simulink library "tetherM_cl"  (R2022a)
settings: Solver=VariableStepAuto  StartTime=0.0  StopTime=10.0  RelTol=1e-3
undefined symbols (not defined in the file): env, initNodePos, nodePosToLinkPos, nodePosToLinkPos_ul, numNodes, tetherReelSpeed, thr, vhcl
libraries: matrix_library x2, firstOrderFilter_ul x1
settings Model: Creator=mr-jo  LastModifiedBy=jbfine
settings SolverCC: AlgebraicLoopSolver=TrustRegion
settings DebuggingCC: UnconnectedInputMsg=warning  UnconnectedOutputMsg=warning  UnconnectedLineMsg=warning  SFMachineParentedDataDiag=warning

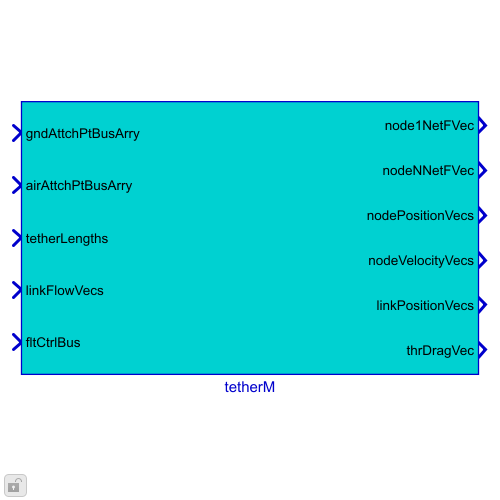
[thumbnail: Simulink's stored preview of the top-level diagram]
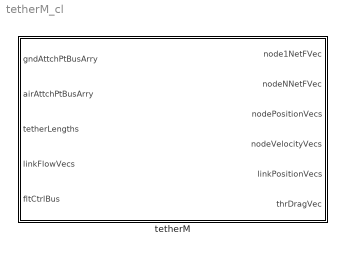
== system tetherM_cl ==
  tetherM : Subsystem  VariantControl=VSS_tethers_tetherM  mask{thr=thr, fluidDensity=env.water.density.Value, gravity=env.gravAccel.Value}
      mask prompts: thr "Tether001 Object"; fluidDensity "Fluid Density"; gravity "Gravitational Aceleration"

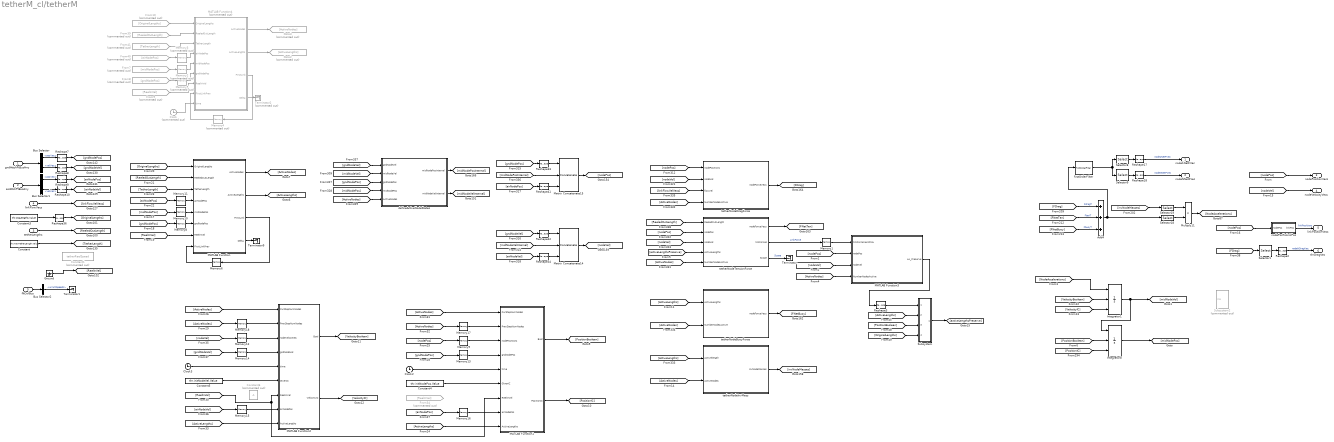
== system tetherM_cl/tetherM ==
  gndAttchPtBusArry : Inport  OutDataTypeStr=Bus: thrAttachPtKinematicsBus
  airAttchPtBusArry : Inport  Port=2  OutDataTypeStr=Bus: thrAttachPtKinematicsBus
  tetherLengths : Inport  Port=3
  linkFlowVecs : Inport  Port=4
  fltCtrlBus : Inport  Port=5
  Add4 : Sum  Inputs=3
  Bus Selector : BusSelector  OutputSignals=posVec,velVec
  Bus Selector1 : BusSelector  OutputSignals=posVec,velVec
  Bus Selector2 : BusSelector  OutputSignals=winchSpeeds
  Clock : Clock  Commented=on
  Clock2 : Clock
  Clock3 : Clock
  Constant : Constant  Value=thr.maxTetherLength.Value
  Constant1 : Constant  Commented=on  Value=tetherReelSpeed
  Constant3 : Constant  Value=thr.orgLengths.Value
  Constant4 : Constant  Value=thr.initNodePos.Value
  Constant5 : Constant  Value=thr.initNodeVel.Value
  Constant6 : Constant  Commented=on  Value=-1
  From10 : From  Commented=on  GotoTag=OriginalLengths
  From34 : From  Commented=on  GotoTag=ReelInVel
  From39 : From  Commented=on  GotoTag=ReeledOutLength
  From40 : From  Commented=on  GotoTag=airNodePos
  From41 : From  Commented=on  GotoTag=TetherLength
  From7 : From  Commented=on  GotoTag=midNodePos
  From8 : From  Commented=on  GotoTag=gndNodePos
  From9 : From  Commented=on  GotoTag=ReelInVel
  Goto2 : Goto  Commented=on  GotoTag=ActiveLengths
  Goto3 : Goto  Commented=on  GotoTag=ActiveNodes
  Ground : Ground
  Integrator1 : Integrator  ExternalReset=rising  InitialConditionSource=external
  Integrator8 : Integrator  ExternalReset=rising  InitialConditionSource=external
  MATLAB Function : MATLAB Function  TreatAsAtomicUnit=on  mask{minLinkLength=thr.minLinkLength.Value, minLinkDeviation=thr.minLinkDeviation.Value}
      mask prompts: minLinkLength "Minimum Link Length"; minLinkDeviation "Minimum Devation to Remove Node"
  MATLAB Function1 : MATLAB Function  TreatAsAtomicUnit=on
  MATLAB Function2 : MATLAB Function  TreatAsAtomicUnit=on
  MATLAB Function3 : MATLAB Function  TreatAsAtomicUnit=on  mask{numNodes=thr.numNodes.Value, thrDiam=thr.diameter.Value, youngsMod=thr.youngsMod.Value, dampingRatio=thr.dampingRatio.Value, mass=vhcl.mass.Value}
      mask prompts: numNodes "Number of Nodes"; thrDiam "Tether Diameter"; youngsMod "Youngs Mod of Tether"; dampingRatio "Total Tether Damping Ratio"; mass "Vehicle Mass for Damping"
  MATLAB Function4 : MATLAB Function  Commented=on  TreatAsAtomicUnit=on  mask{minLinkLength=thr.minLinkLength.Value, minLinkDeviation=thr.minLinkDeviation.Value}
      mask prompts: minLinkLength "Minimum Link Length"; minLinkDeviation "Minimum Devation to Remove Node"
  Matrix Concatenate14 : Concatenate  NumInputs=3  Mode=Multidimensional array  ConcatenateDimension=2
  Matrix Concatenate15 : Concatenate  NumInputs=3  Mode=Multidimensional array  ConcatenateDimension=2
  Memory{1,6,8..18} (13 alike) : Memory
  Memory{2..5} (4 alike) : Memory  Commented=on
  Multiply11 : Product
  Reshape{2,7..10,17..18,33..34,41..42} (11 alike) : Reshape  OutputDimensionality=Column vector (2-D)
  Reshape3 : Reshape  OutputDimensionality=Row vector (2-D)
  Reshape36 : Reshape  OutputDimensionality=Row vector (2-D)
  Selector1 : Selector  NumberOfDimensions=2  InputPortWidth=3  IndexOptions=Select all,Starting index (dialog)  Indices=[1 3],thr.numNodes.Value  OutputSizes=1,1
  Selector18 : Selector  NumberOfDimensions=2  InputPortWidth=3  IndexOptions=Select all,Index vector (dialog)  Indices=[1 3],2:thr.numNodes.Value-1  OutputSizes=1,1
  Selector19 : Selector  NumberOfDimensions=2  InputPortWidth=3  IndexOptions=Select all,Index vector (dialog)  Indices=[1 3],2:thr.numNodes.Value-1  OutputSizes=1,1
  Selector8 : Selector  NumberOfDimensions=2  InputPortWidth=3  IndexOptions=Select all,Index vector (dialog)  Indices=[1 3],1  OutputSizes=1,1
  Selector9 : Selector  NumberOfDimensions=2  InputPortWidth=3  IndexOptions=Select all,Starting index (dialog)  Indices=[1 3],thr.numNodes.Value  OutputSizes=1,1
  Subsystem : Subsystem
  Subsystem2 : Subsystem  Commented=on
  Terminator : Terminator
  Terminator1 : Terminator
  Terminator2 : Terminator  Commented=on
  Terminator9 : Terminator
  defineActiveNodeStates : MATLAB Function  TreatAsAtomicUnit=on
  firstOrderFilter : firstOrderFilter_ul/firstOrderFilter  tau=0.1  ic=0
  nodePosToLinkPos : Subsystem  AncestorBlock=nodePosToLinkPos_ul/nodePosToLinkPos
  tetherNodeBuoyForce : MATLAB Function  TreatAsAtomicUnit=on  mask{fluidDensity=fluidDensity, numNodes=thr.numNodes.Value, thrDiam=thr.diameter.Value, tetherDensity=thr.density.Value, gravity=gravity}
      mask prompts: fluidDensity "Fluid Density"; numNodes "Number of Nodes"; thrDiam "Tether Diameter"; tetherDensity "Tether Density"; gravity "Gravitational Acceleration"
  tetherNodeDragForce : MATLAB Function  TreatAsAtomicUnit=on  mask{flowDensity=fluidDensity, numNodes=thr.numNodes.Value, dragCoeff=thr.dragCoeff.Value, thrDiam=thr.diameter.Value}
      mask prompts: flowDensity "Fluid Density"; numNodes "Number of nodes"; dragCoeff "Drag Coefficient of Tether"; thrDiam "Tether Diameter"
  tetherNodeInvMass : MATLAB Function  TreatAsAtomicUnit=on  mask{numNodes=thr.numNodes.Value, thrDiam=thr.diameter.Value, tetherDensity=thr.density.Value}
      mask prompts: numNodes "Number of nodes"; thrDiam "Tether Diameter"; tetherDensity "Tether Density"
  tetherNodeTensionForce : MATLAB Function  TreatAsAtomicUnit=on  mask{numNodes=thr.numNodes.Value, thrDiam=thr.diameter.Value, youngsMod=thr.youngsMod.Value, dampingRatio=thr.dampingRatio.Value, mass=vhcl.mass.Value, minSoftLength=thr.minSoftLength.Value}
      mask prompts: numNodes "Number of Nodes"; thrDiam "Tether Diameter"; youngsMod "Youngs Modulus of Tether"; dampingRatio "Total Tether Damping Ratio"; mass "Vehicle Mass for Damping"; minSoftLength "Min Link Length for Spring Softening"
  node1NetFVec : Outport  VectorParamsAs1DForOutWhenUnconnected=off
  nodeNNetFVec : Outport  Port=2  VectorParamsAs1DForOutWhenUnconnected=off
  nodePositionVecs : Outport  Port=3  VectorParamsAs1DForOutWhenUnconnected=off
  nodeVelocityVecs : Outport  Port=4  VectorParamsAs1DForOutWhenUnconnected=off
  linkPositionVecs : Outport  Port=5  VectorParamsAs1DForOutWhenUnconnected=off
  thrDragVec : Outport  Port=6  VectorParamsAs1DForOutWhenUnconnected=off
  wires:
  Ground/1 -> [ReelInVel]
  [activeLengthsPreserve] -> tetherNodeTensionForce/4(ActiveLengths)
  Integrator1/1 -> Integrator8/1, [midNodeVel]
  [NodeAccelerations] -> Integrator1/1
  Integrator8/1 -> [midNodePos]
  Clock/1 -> MATLAB Function4/9(time)
  From39/1 -> MATLAB Function4/2(ReeledOutLength)
  MATLAB Function4/1(ActiveNodes) -> Goto3/1
  Memory3/1 -> MATLAB Function4/4(airNodePos)
  From40/1 -> Memory3/1
  MATLAB Function4/3(FirstLink) -> Memory4/1
  Memory2/1 -> MATLAB Function4/5(midNodePos)
  From7/1 -> Memory2/1
  MATLAB Function4/4(Delta) -> Terminator2/1
  From8/1 -> Memory5/1
  Memory5/1 -> MATLAB Function4/6(gndNodePos)
  MATLAB Function4/2(ActiveLengths) -> Goto2/1
  From9/1 -> MATLAB Function4/7(ReelInVel)
  From41/1 -> MATLAB Function4/3(TetherLength)
  From10/1 -> MATLAB Function4/1(OriginalLengths)
  Memory4/1 -> MATLAB Function4/8(FirstLinkPrev)
  MATLAB Function3/1(LA_Preserve) -> Reshape3/1
  tetherNodeTensionForce/2(linkForces) -> Memory1/1  "LinkForce"
  Memory1/1 -> MATLAB Function3/1(linkForceVecsPrev)
  [ActiveNodes] -> MATLAB Function3/4(NumberNodesActive)
  [nodeVel] -> MATLAB Function3/3(nodeVel)
  [nodePos] -> MATLAB Function3/2(nodePos)
  Reshape3/1 -> Subsystem/1(In1)
  [OriginalLengths] -> Subsystem/4(In4)
  [PositionBoolean] -> Subsystem/3(In3)
  [ActiveLengths] -> Subsystem/2(In2)
  Subsystem/1(Out1) -> [activeLengthsPreserve]
  MATLAB Function/4(Delta) -> Terminator9/1
  tetherNodeTensionForce/3(Scope) -> Terminator/1  "Scope"
  [nodeVel] -> tetherNodeTensionForce/3(nodeVel)
  [nodeVel] -> tetherNodeDragForce/2(nodeVel)
  [ReelInVel] -> MATLAB Function1/7(ReelInVel), MATLAB Function2/7(ReelInVel)
  Reshape2/1 -> thrDragVec/1  "nodeNDragVec"
  [FDrag] -> Selector1/1
  Selector1/1 -> Reshape2/1
  Selector18/1 -> Multiply11/2
  Add4/1 -> firstOrderFilter/1, Selector18/1
  firstOrderFilter/1 -> Selector8/1, Selector9/1
  [FNetTen] -> Add4/2  "FtenT"
  Reshape18/1 -> nodeNNetFVec/1  "nodeNNetFVec"
  Reshape17/1 -> node1NetFVec/1  "node1NetFVec"
  [ActiveNodes] -> Memory18/1
  [ActiveNodes] -> Memory17/1
  Constant4/1 -> MATLAB Function1/6(GivenIC)
  MATLAB Function1/1(Bool) -> [PositionBoolean]
  [ActiveNodes] -> MATLAB Function2/1(CurStepNumNodes)
  Memory16/1 -> MATLAB Function1/8(airNodePos)
  Clock2/1 -> MATLAB Function1/5(time)
  MATLAB Function2/2(VelocityIC) -> [VelocityIC]
  Memory13/1 -> MATLAB Function1/4(gndNodePos)
  [airNodeVel] -> Memory15/1
  MATLAB Function1/2(PositionIC) -> [PositionIC]
  Clock3/1 -> MATLAB Function2/5(time)
  [gndNodePos] -> Memory13/1
  Memory17/1 -> MATLAB Function1/2(PrevStepNumNodes)
  [nodeVel] -> Memory12/1
  [gndNodeVel] -> Memory14/1
  Memory18/1 -> MATLAB Function2/2(PrevStepNumNodes)
  Constant5/1 -> MATLAB Function2/6(GivenIC)
  Memory14/1 -> MATLAB Function2/4(gndNodeVel)
  [nodePos] -> Memory9/1
  [ActiveLengths] -> MATLAB Function1/9(ActiveLengths)
  [ActiveNodes] -> MATLAB Function1/1(CurStepNumNodes)
  Memory15/1 -> MATLAB Function2/8(airNodePos)
  [airNodePos] -> Memory16/1
  Memory9/1 -> MATLAB Function1/3(nodePositions)
  MATLAB Function2/1(Bool) -> [VelocityBoolean]
  Memory12/1 -> MATLAB Function2/3(nodeVelocities)
  [ActiveLengths] -> MATLAB Function2/9(ActiveLengths)
  MATLAB Function/2(ActiveLengths) -> [ActiveLengths]
  [midNodePos] -> Memory10/1
  MATLAB Function/1(ActiveNodes) -> [ActiveNodes]
  [ReeledOutLength] -> MATLAB Function/2(ReeledOutLength)
  [ReelInVel] -> MATLAB Function/7(ReelInVel)
  [OriginalLengths] -> MATLAB Function/1(OriginalLengths)
  [airNodePos] -> Memory11/1
  [TetherLength] -> MATLAB Function/3(TetherLength)
  MATLAB Function/3(FirstLink) -> Memory6/1
  Memory8/1 -> MATLAB Function/6(gndNodePos)
  Memory10/1 -> MATLAB Function/5(midNodePos)
  Memory11/1 -> MATLAB Function/4(airNodePos)
  Memory6/1 -> MATLAB Function/8(FirstLinkPrev)
  [gndNodePos] -> Memory8/1
  tetherNodeDragForce/1(nodeForceVecs) -> [FDrag]
  [gndNodeVel] -> Reshape42/1
  [ActiveNodes] -> tetherNodeTensionForce/5(NumberNodesActive)
  tetherNodeInvMass/1(invNodeMasses) -> [invNodeMasses]
  [gndNodePos] -> Reshape33/1
  [airNodePos] -> Reshape41/1
  [midNodePosInternal] -> Matrix Concatenate15/2
  [nodePos] -> tetherNodeDragForce/1(nodePositions)
  [ActiveLengths] -> tetherNodeInvMass/1(Activelength)
  tetherNodeBuoyForce/1(nodeForceVecs) -> [FNetBuoy]
  Reshape42/1 -> Matrix Concatenate14/1
  [ActiveNodes] -> tetherNodeBuoyForce/2(NumberNodesActive)
  Reshape41/1 -> Matrix Concatenate15/3
  Reshape33/1 -> Matrix Concatenate15/1
  [airNodeVel] -> Reshape34/1
  Matrix Concatenate14/1 -> [nodeVel]
  tetherNodeTensionForce/1(nodeForceVecs) -> [FNetTen]
  Matrix Concatenate15/1 -> [nodePos]
  [gndNodeVel] -> defineActiveNodeStates/1(gndNodeVel)
  [midNodePos] -> defineActiveNodeStates/4(midNodePos)
  [ActiveNodes] -> defineActiveNodeStates/5(ActiveNodes)
  [midNodeVelInternal] -> Matrix Concatenate14/2
  [gndNodePos] -> defineActiveNodeStates/3(gndNodePos)
  Reshape34/1 -> Matrix Concatenate14/3
  [ActiveNodes] -> tetherNodeDragForce/4(NumberNodesActive)
  [ReeledOutLength] -> tetherNodeTensionForce/1(ReeledOutLength)
  defineActiveNodeStates/2(midNodeVelInternal) -> [midNodeVelInternal]
  [nodePos] -> tetherNodeTensionForce/2(nodePos)
  [midNodeVel] -> defineActiveNodeStates/2(midNodeVel)
  [linkFlowVelVecs] -> tetherNodeDragForce/3(flowVel)
  tetherLengths/1 -> [ReeledOutLength]
  Reshape36/1 -> [OriginalLengths]
  linkFlowVecs/1 -> [linkFlowVelVecs]
  Constant/1 -> [TetherLength]
  defineActiveNodeStates/1(midNodePosInternal) -> [midNodePosInternal]
  [invNodeMasses] -> Selector19/1
  Selector19/1 -> Multiply11/1
  [FDrag] -> Add4/1  "FdragT"
  Multiply11/1 -> [NodeAccelerations]
  [FNetBuoy] -> Add4/3  "FbuoyT"
  [PositionIC] -> Integrator8/3
  Selector8/1 -> Reshape17/1
  Selector9/1 -> Reshape18/1
  [PositionBoolean] -> Integrator8/2
  [VelocityIC] -> Integrator1/3
  [VelocityBoolean] -> Integrator1/2
  [ActiveLengths] -> tetherNodeBuoyForce/1(ActiveLengths)
  [ActiveNodes] -> tetherNodeInvMass/2(ActiveNodes)
  Bus Selector1/2 -> Reshape10/1  "<velVec>"
  gndAttchPtBusArry/1 -> Bus Selector/1
  Reshape7/1 -> [gndNodePos]
  Reshape10/1 -> [airNodeVel]
  Reshape9/1 -> [airNodePos]
  airAttchPtBusArry/1 -> Bus Selector1/1
  Bus Selector/2 -> Reshape8/1  "<velVec>"
  Bus Selector1/1 -> Reshape9/1  "<posVec>"
  Reshape8/1 -> [gndNodeVel]
  Bus Selector/1 -> Reshape7/1  "<posVec>"
  Constant3/1 -> Reshape36/1
  [nodePos] -> nodePositionVecs/1
  [nodeVel] -> nodeVelocityVecs/1
  nodePosToLinkPos/1("linkPos ") -> linkPositionVecs/1  "linkPositions"
  [nodePos] -> nodePosToLinkPos/1("nodePos ")
  fltCtrlBus/1 -> Bus Selector2/1
  Bus Selector2/1 -> Terminator1/1  "<winchSpeeds>"

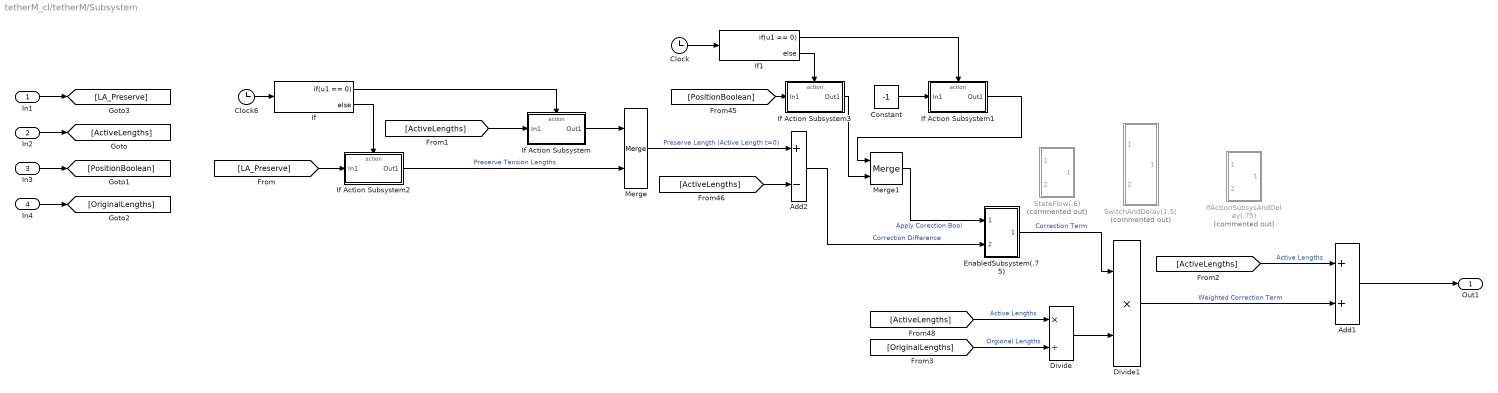
== system tetherM_cl/tetherM/Subsystem ==
  In1 : Inport
  In2 : Inport  Port=2
  In3 : Inport  Port=3
  In4 : Inport  Port=4
  Add1 : Sum
  Add2 : Sum  Inputs=+-
  Clock : Clock
  Clock6 : Clock
  Constant : Constant  Value=-1
  Divide : Product  Inputs=*/
  Divide1 : Product  Inputs=**
  EnabledSubsystem(.75) : Subsystem
  If : If  IfExpression=u1 == 0
  If Action Subsystem : Subsystem  TreatAsAtomicUnit=on
  If Action Subsystem1 : Subsystem  TreatAsAtomicUnit=on
  If Action Subsystem2 : Subsystem  TreatAsAtomicUnit=on
  If Action Subsystem3 : Subsystem  TreatAsAtomicUnit=on
  If1 : If  IfExpression=u1 == 0
  IfActionSubsysAndDelay(.75) : Subsystem  Commented=on
  Merge : Merge  InitialOutput=thr.orgLengths.Value
  Merge1 : Merge  InitialOutput=[-1]
  StateFlow(.6) : Subsystem  Commented=on
  SwitchAndDelay(1.5) : Subsystem  Commented=on
  Out1 : Outport
  wires:
  Add1/1 -> Out1/1
  [ActiveLengths] -> Add1/1  "Active Lengths"
  [ActiveLengths] -> Divide/1  "Active Lengths"
  [ActiveLengths] -> Add2/2
  [ActiveLengths] -> If Action Subsystem/1(In1)
  If Action Subsystem1/1(Out1) -> Merge1/1
  Constant/1 -> If Action Subsystem1/1(In1)
  If Action Subsystem3/1(Out1) -> Merge1/2
  Merge1/1 -> EnabledSubsystem(.75)/1(Enable)  "Apply Corection Bool"
  If1/2 -> If Action Subsystem3/Action
  If1/1 -> If Action Subsystem1/Action
  Clock/1 -> If1/1
  EnabledSubsystem(.75)/1(Out1) -> Divide1/1  "Correction Term"
  Add2/1 -> EnabledSubsystem(.75)/2(In2)  "Correction Difference"
  [PositionBoolean] -> If Action Subsystem3/1(In1)
  Merge/1 -> Add2/1  "Preserve Length (Active Length t=0)"
  [LA_Preserve] -> If Action Subsystem2/1(In1)
  In4/1 -> [OriginalLengths]
  In3/1 -> [PositionBoolean]
  In2/1 -> [ActiveLengths]
  In1/1 -> [LA_Preserve]
  If/1 -> If Action Subsystem/Action
  Divide/1 -> Divide1/2
  If/2 -> If Action Subsystem2/Action
  If Action Subsystem/1(Out1) -> Merge/1
  [OriginalLengths] -> Divide/2  "Orgional Lengths"
  If Action Subsystem2/1(Out1) -> Merge/2  "Preserve Tension Lengths"
  Clock6/1 -> If/1
  Divide1/1 -> Add1/2  "Weighted Correction Term"

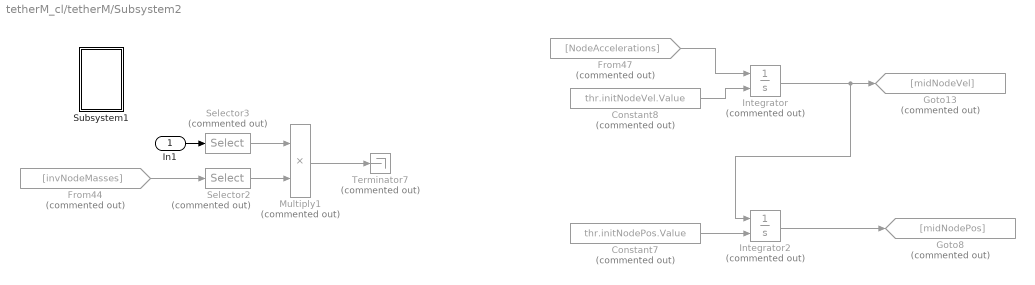
== system tetherM_cl/tetherM/Subsystem2 ==
  In1 : Inport
  Constant7 : Constant  Commented=on  Value=thr.initNodePos.Value
  Constant8 : Constant  Commented=on  Value=thr.initNodeVel.Value
  From44 : From  Commented=on  GotoTag=invNodeMasses
  From47 : From  Commented=on  GotoTag=NodeAccelerations
  Goto13 : Goto  Commented=on  GotoTag=midNodeVel
  Goto8 : Goto  Commented=on  GotoTag=midNodePos
  Integrator : Integrator  Commented=on  InitialConditionSource=external
  Integrator2 : Integrator  Commented=on  InitialConditionSource=external
  Multiply1 : Product  Commented=on
  Selector2 : Selector  Commented=on  NumberOfDimensions=2  InputPortWidth=3  IndexOptions=Select all,Index vector (dialog)  Indices=[1 3],2:thr.numNodes.Value-1  OutputSizes=1,1
  Selector3 : Selector  Commented=on  NumberOfDimensions=2  InputPortWidth=3  IndexOptions=Select all,Index vector (dialog)  Indices=[1 3],2:thr.numNodes.Value-1  OutputSizes=1,1
  Subsystem1 : Subsystem
  Terminator7 : Terminator  Commented=on
  wires:
  In1/1 -> Selector3/1
  Selector2/1 -> Multiply1/2
  From44/1 -> Selector2/1
  Integrator2/1 -> Goto8/1
  Constant8/1 -> Integrator/2
  Multiply1/1 -> Terminator7/1
  From47/1 -> Integrator/1
  Constant7/1 -> Integrator2/2
  Integrator/1 -> Goto13/1, Integrator2/1
  Selector3/1 -> Multiply1/1

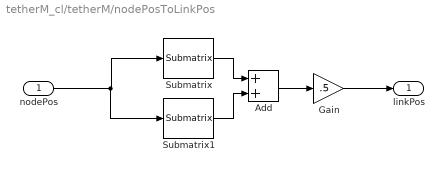
== system tetherM_cl/tetherM/nodePosToLinkPos ==
  "nodePos " : Inport
  Add : Sum
  Gain : Gain  Gain=.5
  Submatrix : matrix_library/Submatrix  RowSpan=All rows  RowStartMode=First  RowStartIndex=1  RowEndMode=Last  RowEndIndex=1  ColSpan=Range of columns  ColStartMode=First  ColStartIndex=1  ColEndMode=Offset from last  ColEndIndex=1
      settings: SourceProductBaseCode=SL
  Submatrix1 : matrix_library/Submatrix  RowSpan=All rows  RowStartMode=First  RowStartIndex=1  RowEndMode=Last  RowEndIndex=1  ColSpan=Range of columns  ColStartMode=Index  ColStartIndex=2  ColEndMode=Last  ColEndIndex=1
      settings: SourceProductBaseCode=SL
  "linkPos " : Outport  VectorParamsAs1DForOutWhenUnconnected=off
  wires:
  "nodePos "/1 -> Submatrix1/1, Submatrix/1
  Gain/1 -> "linkPos "/1
  Add/1 -> Gain/1
  Submatrix/1 -> Add/1
  Submatrix1/1 -> Add/2

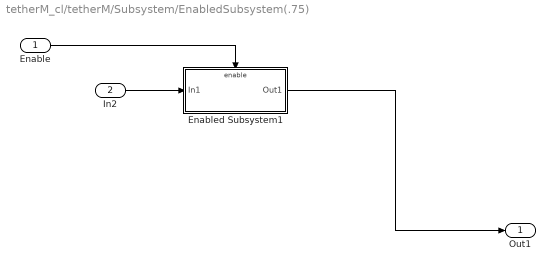
== system tetherM_cl/tetherM/Subsystem/EnabledSubsystem(.75) ==
  Enable : Inport
  In2 : Inport  Port=2
  Enabled Subsystem1 : Subsystem  TreatAsAtomicUnit=on
  Out1 : Outport
  wires:
  In2/1 -> Enabled Subsystem1/1(In1)
  Enabled Subsystem1/1(Out1) -> Out1/1
  Enable/1 -> Enabled Subsystem1/Enable

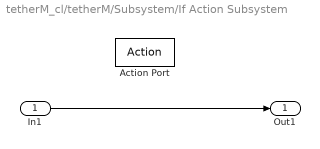
== system tetherM_cl/tetherM/Subsystem/If Action Subsystem ==
  In1 : Inport
  Action Port : ActionPort
  Out1 : Outport
  wires:
  In1/1 -> Out1/1

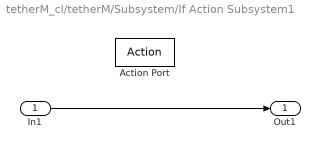
== system tetherM_cl/tetherM/Subsystem/If Action Subsystem1 ==
  In1 : Inport
  Action Port : ActionPort
  Out1 : Outport
  wires:
  In1/1 -> Out1/1

== system tetherM_cl/tetherM/Subsystem/If Action Subsystem2 ==
  In1 : Inport
  Action Port : ActionPort
  Out1 : Outport
  wires:
  In1/1 -> Out1/1

== system tetherM_cl/tetherM/Subsystem/If Action Subsystem3 ==
  In1 : Inport
  Action Port : ActionPort
  Out1 : Outport
  wires:
  In1/1 -> Out1/1

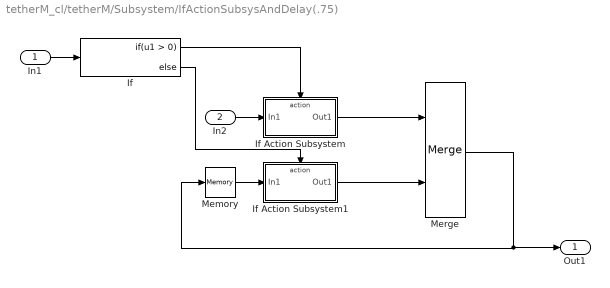
== system tetherM_cl/tetherM/Subsystem/IfActionSubsysAndDelay(.75) ==
  In1 : Inport
  In2 : Inport  Port=2
  If : If
  If Action Subsystem : Subsystem  TreatAsAtomicUnit=on
  If Action Subsystem1 : Subsystem  TreatAsAtomicUnit=on
  Memory : Memory
  Merge : Merge  InitialOutput=thr.orgLengths.Value
  Out1 : Outport
  wires:
  In2/1 -> If Action Subsystem/1(In1)
  In1/1 -> If/1
  Merge/1 -> Memory/1, Out1/1
  Memory/1 -> If Action Subsystem1/1(In1)
  If Action Subsystem1/1(Out1) -> Merge/2
  If Action Subsystem/1(Out1) -> Merge/1
  If/1 -> If Action Subsystem/Action
  If/2 -> If Action Subsystem1/Action

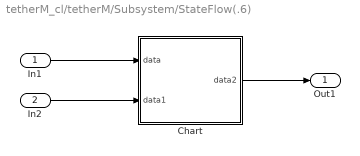
== system tetherM_cl/tetherM/Subsystem/StateFlow(.6) ==
  In1 : Inport
  In2 : Inport  Port=2
  Chart : Stateflow chart  TreatAsAtomicUnit=on
  Out1 : Outport
  wires:
  Chart/1(data2) -> Out1/1
  In2/1 -> Chart/2(data1)
  In1/1 -> Chart/1(data)

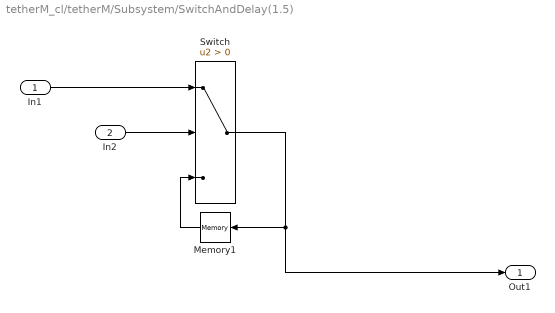
== system tetherM_cl/tetherM/Subsystem/SwitchAndDelay(1.5) ==
  In1 : Inport
  In2 : Inport  Port=2
  Memory1 : Memory  InitialCondition=zeros(size(thr.orgLengths.Value))
  Switch : Switch  Criteria=u2 > Threshold  SaturateOnIntegerOverflow=off  InputSameDT=off
  Out1 : Outport
  wires:
  In1/1 -> Switch/1
  In2/1 -> Switch/2
  Memory1/1 -> Switch/3
  Switch/1 -> Memory1/1, Out1/1

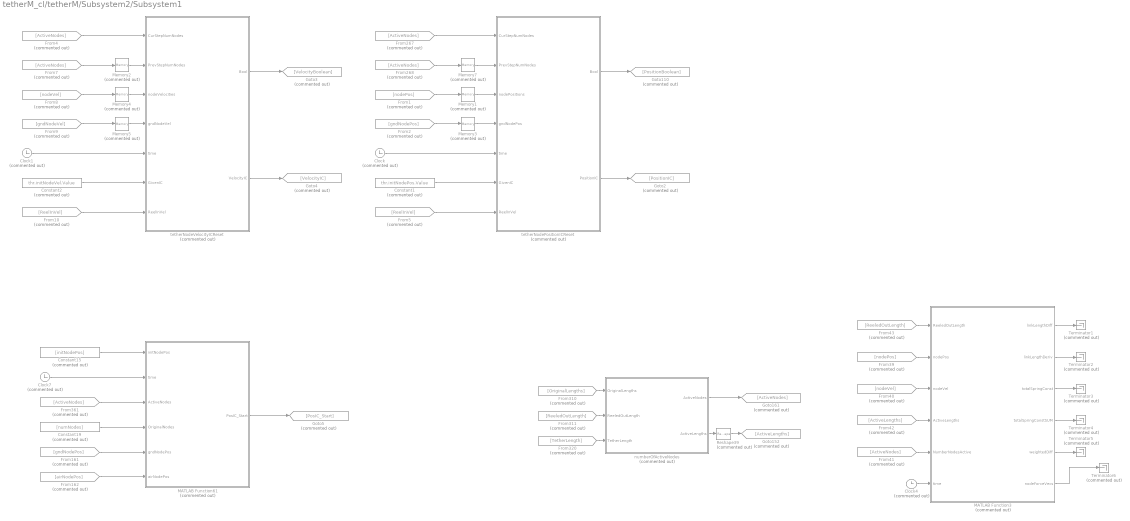
== system tetherM_cl/tetherM/Subsystem2/Subsystem1 ==
  Clock{,1,4,7} (4 alike) : Clock  Commented=on
  Constant1 : Constant  Commented=on  Value=thr.initNodePos.Value
  Constant15 : Constant  Commented=on  Value=[initNodePos]
  Constant19 : Constant  Commented=on  Value=[numNodes]
  Constant2 : Constant  Commented=on  Value=thr.initNodeVel.Value
  From1 : From  Commented=on  GotoTag=nodePos
  From10 : From  Commented=on  GotoTag=ReelInVel
  From161 : From  Commented=on  GotoTag=gndNodePos
  From162 : From  Commented=on  GotoTag=airNodePos
  From2 : From  Commented=on  GotoTag=gndNodePos
  From{4,7,41,267..268,361} (6 alike) : From  Commented=on  GotoTag=ActiveNodes
  From310 : From  Commented=on  GotoTag=OriginalLengths
  From311 : From  Commented=on  GotoTag=ReeledOutLength
  From320 : From  Commented=on  GotoTag=TetherLength
  From39 : From  Commented=on  GotoTag=nodePos
  From40 : From  Commented=on  GotoTag=nodeVel
  From42 : From  Commented=on  GotoTag=ActiveLengths
  From43 : From  Commented=on  GotoTag=ReeledOutLength
  From5 : From  Commented=on  GotoTag=ReelInVel
  From8 : From  Commented=on  GotoTag=nodeVel
  From9 : From  Commented=on  GotoTag=gndNodeVel
  Goto110 : Goto  Commented=on  GotoTag=PositionBoolean
  Goto152 : Goto  Commented=on  GotoTag=ActiveLengths
  Goto161 : Goto  Commented=on  GotoTag=ActiveNodes
  Goto2 : Goto  Commented=on  GotoTag=PositionIC
  Goto3 : Goto  Commented=on  GotoTag=VelocityBoolean
  Goto4 : Goto  Commented=on  GotoTag=VelocityIC
  Goto5 : Goto  Commented=on  GotoTag=PosIC_Start
  MATLAB Function3 : MATLAB Function  Commented=on  TreatAsAtomicUnit=on  mask{numNodes=thr.numNodes.Value, thrDiam=thr.diameter.Value, youngsMod=thr.youngsMod.Value, dampingRatio=thr.dampingRatio.Value, mass=thr.vehicleMass.Value}
      mask prompts: numNodes "Number of Nodes"; thrDiam "Tether Diameter"; youngsMod "Youngs Modulus of Tether"; dampingRatio "Total Tether Damping Ratio"; mass "Vehicle Mass for Damping"
  MATLAB Function61 : MATLAB Function  Commented=on  TreatAsAtomicUnit=on
  Memory{1..5,7} (6 alike) : Memory  Commented=on
  Reshape39 : Reshape  Commented=on  OutputDimensionality=Row vector (2-D)
  Terminator{1..6} (6 alike) : Terminator  Commented=on
  numberOfActiveNodes : MATLAB Function  Commented=on  TreatAsAtomicUnit=on
  tetherNodePositionICReset : MATLAB Function  Commented=on  TreatAsAtomicUnit=on
  tetherNodeVelocityICReset : MATLAB Function  Commented=on  TreatAsAtomicUnit=on
  wires:
  numberOfActiveNodes/2(ActiveLengths) -> Reshape39/1
  MATLAB Function61/1(PosIC_Start) -> Goto5/1
  From311/1 -> numberOfActiveNodes/2(ReeledOutLength)
  From268/1 -> Memory7/1
  tetherNodePositionICReset/2(PositionIC) -> Goto2/1
  From310/1 -> numberOfActiveNodes/1(OriginalLengths)
  From2/1 -> Memory3/1
  From10/1 -> tetherNodeVelocityICReset/7(ReelInVel)
  From4/1 -> tetherNodeVelocityICReset/1(CurStepNumNodes)
  tetherNodeVelocityICReset/2(VelocityIC) -> Goto4/1
  From320/1 -> numberOfActiveNodes/3(TetherLength)
  From5/1 -> tetherNodePositionICReset/7(ReelInVel)
  Clock1/1 -> tetherNodeVelocityICReset/5(time)
  From8/1 -> Memory4/1
  Constant1/1 -> tetherNodePositionICReset/6(GivenIC)
  Clock7/1 -> MATLAB Function61/2(time)
  From162/1 -> MATLAB Function61/6(airNodePos)
  Memory3/1 -> tetherNodePositionICReset/4(gndNodePos)
  Constant19/1 -> MATLAB Function61/4(OriginalNodes)
  MATLAB Function3/1(linkLengthDiff) -> Terminator1/1
  From161/1 -> MATLAB Function61/5(gndNodePos)
  MATLAB Function3/5(weightedDiff) -> Terminator5/1
  Constant2/1 -> tetherNodeVelocityICReset/6(GivenIC)
  tetherNodePositionICReset/1(Bool) -> Goto110/1
  MATLAB Function3/6(nodeForceVecs) -> Terminator6/1
  From9/1 -> Memory5/1
  Memory5/1 -> tetherNodeVelocityICReset/4(gndNodeVel)
  Memory7/1 -> tetherNodePositionICReset/2(PrevStepNumNodes)
  From7/1 -> Memory2/1
  numberOfActiveNodes/1(ActiveNodes) -> Goto161/1
  Clock/1 -> tetherNodePositionICReset/5(time)
  Memory1/1 -> tetherNodePositionICReset/3(nodePositions)
  Clock4/1 -> MATLAB Function3/6(time)
  Reshape39/1 -> Goto152/1
  From43/1 -> MATLAB Function3/1(ReeledOutLength)
  MATLAB Function3/2(linkLengthDeriv) -> Terminator2/1
  From267/1 -> tetherNodePositionICReset/1(CurStepNumNodes)
  MATLAB Function3/4(totalSpringConstSUM) -> Terminator4/1
  Memory4/1 -> tetherNodeVelocityICReset/3(nodeVelocities)
  From41/1 -> MATLAB Function3/5(NumberNodesActive)
  From1/1 -> Memory1/1
  MATLAB Function3/3(totalSpringConst) -> Terminator3/1
  From42/1 -> MATLAB Function3/4(ActiveLengths)
  tetherNodeVelocityICReset/1(Bool) -> Goto3/1
  From361/1 -> MATLAB Function61/3(ActiveNodes)
  From39/1 -> MATLAB Function3/2(nodePos)
  Memory2/1 -> tetherNodeVelocityICReset/2(PrevStepNumNodes)
  From40/1 -> MATLAB Function3/3(nodeVel)
  Constant15/1 -> MATLAB Function61/1(initNodePos)

== system tetherM_cl/tetherM/Subsystem/EnabledSubsystem(.75)/Enabled Subsystem1 ==
  In1 : Inport
  Enable : EnablePort
  Out1 : Outport  InitialOutput=zeros(size(thr.orgLengths.Value))
  wires:
  In1/1 -> Out1/1

== system tetherM_cl/tetherM/Subsystem/IfActionSubsysAndDelay(.75)/If Action Subsystem ==
  In1 : Inport
  Action Port : ActionPort
  Out1 : Outport
  wires:
  In1/1 -> Out1/1

== system tetherM_cl/tetherM/Subsystem/IfActionSubsysAndDelay(.75)/If Action Subsystem1 ==
  In1 : Inport
  Action Port : ActionPort
  Out1 : Outport
  wires:
  In1/1 -> Out1/1

== stateflow chart tetherM_cl/tetherM/Subsystem/StateFlow(.6)/Chart ==
  (default) -> (junction 4) : [data>0]{data2=data1;}
  data: data input; data1 input; data2 output

== matlab function tetherM_cl/tetherM/Subsystem2/Subsystem1/MATLAB Function3 ==
  data: ReeledOutLength input; linkLengthDiff output; nodePos input; linkLengthDeriv output; totalSpringConst output; nodeVel input; ActiveLengths input; NumberNodesActive input; time input; numNodes parameter; totalSpringConstSUM output; thrDiam parameter; youngsMod parameter; dampingRatio parameter; mass parameter; weightedDiff output; nodeForceVecs output
function [linkLengthDiff,linkLengthDeriv,totalSpringConst,totalSpringConstSUM,weightedDiff,nodeForceVecs] = fcn(ReeledOutLength, nodePos,nodeVel,ActiveLengths,NumberNodesActive,time, numNodes, thrDiam, youngsMod, dampingRatio, mass)

No = numNodes;
Na = NumberNodesActive;

unstretchedLength = ReeledOutLength; %Total Reeled out length

%finds vectors between nodes
linkVecs  = diff(nodePos,1,2);
linkLength = sqrt(sum(linkVecs.^2));

%Finds unit vectors between nodes
linkUnitVecs = zeros(3,numNodes-1);
linkUnitVecs(1:3,(No-Na+1):end) = linkVecs(1:3,(No-Na+1):end)./repmat(sqrt(sum((linkVecs(1:3,(No-Na+1):end).^2),1)),[3 1]);

%prevent divide by zero if reeled in 
linkUnitVecs(isnan(linkUnitVecs))=0;

%Rate of change of all links
linkLengthDeriv = dot(nodeVel(:,2:end)-nodeVel(:,1:end-1),linkUnitVecs);
linkLengthDiff = (linkLength-ActiveLengths);


%Tension through jump

totalSpringConst = youngsMod*(pi/4)*(thrDiam^2)/unstretchedLength;
%Finds Spring Constant
SpringConsts = zeros(1,numNodes-1);
if Na>2
    SpringConsts(:,(No-Na+2):end) = youngsMod*(pi/4)*(thrDiam^2)./ActiveLengths(1,(end-Na+3):end);
%     if ActiveLengths(1,(end-Na+2))>minSoftLength
         SpringConsts(:,(No-Na+1)) = youngsMod*(pi/4)*(thrDiam^2)./ActiveLengths(1,(end-Na+2));
%     else %If below spring softening limit
%        SpringConsts(:,(No-Na+1)) = youngsMod*(pi/4)*(thrDiam^2)./minSoftLength;
%     end
else %If on last link
    SpringConsts(end) = totalSpringConst;
end

oneOverSpringSUM = 0;
for ii = (No-Na+1):(No)-1
    oneOverSpringSUM = oneOverSpringSUM + 1/SpringConsts(1,ii);
end
totalSpringConstSUM = 1/oneOverSpringSUM;

weightedDiff =  linkLengthDiff/sum(linkLengthDiff);

springForce = SpringConsts.*linkLengthDiff;

totalLinkForceVec = repmat(springForce,[3 1]).*linkUnitVecs;

nodeForceVecs = zeros(3,No);
nodeForceVecs(:,(No-Na+1):end) = [totalLinkForceVec(:,(No-Na+1)) diff(totalLinkForceVec(:,(No-Na+1):end),1,2) -totalLinkForceVec(:,end)];
%nodeForceVecs = [totalLinkForceVec(:,1) diff(totalLinkForceVec,1,2) -totalLinkForceVec(:,end)];

%Moves Reeled in bottom  node force to Ground Node
if SpringConsts(1) == 0
    nodeForceVecs(:,1) = nodeForceVecs(:,No-Na+1);
    nodeForceVecs(:,No-Na+1) = [0;0;0];
end

end

== matlab function tetherM_cl/tetherM/Subsystem2/Subsystem1/MATLAB Function61 ==
  data: initNodePos input size=[3,numNodes-2]; time input size=1; ActiveNodes input size=1; OriginalNodes input size=1; gndNodePos input size=[3,1]; airNodePos input size=[3,1]; PosIC_Start output
function PosIC_Start = fcn(initNodePos,time, ActiveNodes, OriginalNodes,gndNodePos,airNodePos)

if time==0
    Na = ActiveNodes;
    No = 11;%OriginalNodes;
    
    TetherVec = [linspace(gndNodePos(1),airNodePos(1),Na);...
                 linspace(gndNodePos(2),airNodePos(2),Na);...
                 linspace(gndNodePos(3),airNodePos(3),Na)];
    PosIC_Start = [gndNodePos(1)*ones(1,No-2);...
             gndNodePos(2)*ones(1,No-2);...
             gndNodePos(3)*ones(1,No-2)];

    % initNodePos   
    PosIC_Start(1,((No-Na)+1):end) = linspace(TetherVec(1,2),TetherVec(1,end-1),Na-2);
    PosIC_Start(2,((No-Na)+1):end) = linspace(TetherVec(2,2),TetherVec(2,end-1),Na-2);
    PosIC_Start(3,((No-Na)+1):end) = linspace(TetherVec(3,2),TetherVec(3,end-1),Na-2);
else
    PosIC_Start = zeros(3,size(initNodePos,2));
end

== matlab function tetherM_cl/tetherM/Subsystem2/Subsystem1/numberOfActiveNodes ==
  data: OriginalLengths input; ActiveNodes output; ReeledOutLength input; ActiveLengths output; TetherLength input
function [ActiveNodes, ActiveLengths] = fcn(OriginalLengths, ReeledOutLength, TetherLength)
    [ActiveNodes, ActiveLengths] = numberOfActiveNodes(OriginalLengths, ReeledOutLength, TetherLength);
end

== matlab function tetherM_cl/tetherM/Subsystem2/Subsystem1/tetherNodePositionICReset ==
  data: CurStepNumNodes input; Bool output; PrevStepNumNodes input; nodePositions input; gndNodePos input; PositionIC output; time input; GivenIC input; ReelInVel input
function [Bool,PositionIC]  = fcn(CurStepNumNodes, PrevStepNumNodes, nodePositions, gndNodePos, time, GivenIC, ReelInVel)
    [Bool,PositionIC]  = tetherNodePositionICReset(CurStepNumNodes, PrevStepNumNodes, nodePositions, gndNodePos, time, GivenIC, ReelInVel);
end

== matlab function tetherM_cl/tetherM/Subsystem2/Subsystem1/tetherNodeVelocityICReset ==
  data: CurStepNumNodes input; Bool output; PrevStepNumNodes input; nodeVelocities input; gndNodeVel input; time input; GivenIC input; ReelInVel input; VelocityIC output
function [Bool,VelocityIC]  = fcn(CurStepNumNodes, PrevStepNumNodes, nodeVelocities, gndNodeVel, time, GivenIC, ReelInVel)
    [Bool,VelocityIC]  = tetherNodeVelocityICReset(CurStepNumNodes, PrevStepNumNodes, nodeVelocities, gndNodeVel, time, GivenIC, ReelInVel);
end

== matlab function tetherM_cl/tetherM/defineActiveNodeStates ==
  data: gndNodeVel input size=[3,1]; midNodeVel input size=[3,thr.numNodes.Value-2]; gndNodePos input size=[3,1]; midNodePosInternal output size=[3,thr.numNodes.Value-2]; midNodePos input size=[3,thr.numNodes.Value-2]; ActiveNodes input size=1; midNodeVelInternal output size=[3,thr.numNodes.Value-2]
function [midNodePosInternal,  midNodeVelInternal] = fcn(gndNodeVel,midNodeVel,gndNodePos, midNodePos, ActiveNodes)

No = size(midNodePos,2)+2;
Na = ActiveNodes;

% Reeled In Nodes are ground
midNodePosInternal = [gndNodePos(1)*ones(1,No-2);...
                      gndNodePos(2)*ones(1,No-2);...
                      gndNodePos(3)*ones(1,No-2)];
                  
midNodeVelInternal = [gndNodeVel(1)*ones(1,No-2);...
                      gndNodeVel(2)*ones(1,No-2);...
                      gndNodeVel(3)*ones(1,No-2)];              
                  
% Given for unalternd nodes
midNodePosInternal(:,((No-Na)+1):end) = midNodePos(:,((No-Na)+1):end);
midNodeVelInternal(:,((No-Na)+1):end) = midNodeVel(:,((No-Na)+1):end);

== matlab function tetherM_cl/tetherM/tetherNodeBuoyForce ==
  data: ActiveLengths input; NumberNodesActive input; nodeForceVecs output size=[3,thr.numNodes.Value]; numNodes parameter; thrDiam parameter; tetherDensity parameter; gravity parameter; fluidDensity parameter
function nodeForceVecs = fcn(ActiveLengths, NumberNodesActive, numNodes, thrDiam, tetherDensity, gravity, fluidDensity)
    nodeForceVecs = tetherNodeBuoyForce(ActiveLengths, NumberNodesActive, numNodes, thrDiam, tetherDensity, gravity, fluidDensity);
end

== matlab function tetherM_cl/tetherM/tetherNodeDragForce ==
  data: nodePositions input size=[3,thr.numNodes.Value]; nodeVel input size=[3,thr.numNodes.Value]; flowVel input size=[3,thr.numNodes.Value-1]; NumberNodesActive input size=1; nodeForceVecs output size=[3,thr.numNodes.Value]; numNodes parameter size=1; dragCoeff parameter; thrDiam parameter; flowDensity parameter
function nodeForceVecs = fcn(nodePositions,nodeVel, flowVel, NumberNodesActive, numNodes, dragCoeff, thrDiam, flowDensity)
    nodeForceVecs = tetherNodeDragForce(nodePositions,nodeVel, flowVel, NumberNodesActive, numNodes, dragCoeff, thrDiam, flowDensity);
end

== matlab function tetherM_cl/tetherM/tetherNodeInvMass ==
  data: invNodeMasses output size=[3,thr.numNodes.Value]; Activelength input; ActiveNodes input; numNodes parameter; thrDiam parameter; tetherDensity parameter
function invNodeMasses  = fcn(Activelength,ActiveNodes, numNodes, thrDiam, tetherDensity)
    invNodeMasses  = tetherNodeInvMass(Activelength,ActiveNodes, numNodes, thrDiam, tetherDensity);
end

== matlab function tetherM_cl/tetherM/tetherNodeTensionForce ==
  data: ReeledOutLength input; nodePos input; nodeForceVecs output size=[3,thr.numNodes.Value]; linkForces output; nodeVel input; ActiveLengths input; NumberNodesActive input; numNodes parameter; thrDiam parameter; youngsMod parameter; dampingRatio parameter; mass parameter; minSoftLength parameter; Scope output size=[1,thr.numNodes.Value-1]
function  [nodeForceVecs,linkForces,Scope]    = fcn(ReeledOutLength, nodePos, nodeVel, ActiveLengths,NumberNodesActive, numNodes, thrDiam, youngsMod, dampingRatio, mass,minSoftLength)
     [nodeForceVecs,linkForces,Scope]  = tetherNodeTensionForce(ReeledOutLength, nodePos, nodeVel, ActiveLengths,NumberNodesActive, numNodes, thrDiam, youngsMod, dampingRatio, mass,minSoftLength);
    Scope;
end

== matlab function tetherM_cl/tetherM/MATLAB Function ==
  data: OriginalLengths input; ActiveNodes output; ReeledOutLength input; TetherLength input; airNodePos input; midNodePos input; gndNodePos input; ReelInVel input; FirstLinkPrev input; ActiveLengths output size=[1,thr.numNodes.Value-1]; FirstLink output; minLinkLength parameter; minLinkDeviation parameter; Delta output
function [ActiveNodes, ActiveLengths,FirstLink,Delta] = fcn(OriginalLengths, ReeledOutLength, TetherLength,airNodePos, midNodePos, gndNodePos,ReelInVel,FirstLinkPrev,minLinkLength, minLinkDeviation)
    [ActiveNodes, ActiveLengths,FirstLink,Delta] = numberOfActiveNodes(OriginalLengths, ReeledOutLength, TetherLength,airNodePos, midNodePos, gndNodePos,ReelInVel,FirstLinkPrev,minLinkLength,minLinkDeviation);
end

== matlab function tetherM_cl/tetherM/MATLAB Function1 ==
  data: CurStepNumNodes input; Bool output; PrevStepNumNodes input; nodePositions input; gndNodePos input; time input; GivenIC input; ReelInVel input; airNodePos input; ActiveLengths input; PositionIC output
function [Bool,PositionIC]  = fcn(CurStepNumNodes, PrevStepNumNodes, nodePositions, gndNodePos, time, GivenIC, ReelInVel, airNodePos, ActiveLengths)

if ReelInVel<=0
    if time==0
        PositionIC = GivenIC;
        Bool = 1;
    else
        Na = CurStepNumNodes;
        No = size(nodePositions,2);

        if PrevStepNumNodes==0
            Nc = CurStepNumNodes;
            Np = Nc;
        else
            Np = PrevStepNumNodes;
            Nc = CurStepNumNodes;
        end

        PositionIC = [gndNodePos(1)*ones(1,No-2);...
                      gndNodePos(2)*ones(1,No-2);...
                      gndNodePos(3)*ones(1,No-2)];
        if Nc == Np
            Bool = -1;
        else
            Bool = 1;
            PositionIC(:,(No-Na+1):end) = nodePositions(:,(No-Na+2):end-1);
        end
    end         
else
    if time==0
        PositionIC = GivenIC;
        Bool = 1;
    else
        Na = CurStepNumNodes;
        No = size(nodePositions,2);

        if PrevStepNumNodes==0
            Nc = CurStepNumNodes;
            Np = Nc;
        else
            Np = PrevStepNumNodes;
            Nc = CurStepNumNodes;
        end

        PositionIC = [gndNodePos(1)*ones(1,No-2);...
                      gndNodePos(2)*ones(1,No-2);...
                      gndNodePos(3)*ones(1,No-2)];
        if Nc == Np
            Bool = -1;
        else
            Bool = 1;
            linkVecs  = diff(nodePositions,1,2);
            linkVecsUnit = linkVecs./repmat(sqrt(sum((linkVecs.^2),1)),[3 1]);
            linkVecsUnit(isnan(linkVecsUnit))=0;
            PositionIC(:,(No-Na+2):end) = nodePositions(:,(No-Na+3):end-1);
            PositionIC(:,(No-Na+1)) = linkVecsUnit(:,(No-Na+1)).*ActiveLengths(:,No-Na+1);
        end
    end
end

== matlab function tetherM_cl/tetherM/MATLAB Function2 ==
  data: CurStepNumNodes input; Bool output; PrevStepNumNodes input; nodeVelocities input; gndNodeVel input; time input; GivenIC input; ReelInVel input; airNodePos input; ActiveLengths input; VelocityIC output
function [Bool,VelocityIC]  = fcn(CurStepNumNodes, PrevStepNumNodes, nodeVelocities, gndNodeVel, time, GivenIC, ReelInVel, airNodePos, ActiveLengths)

if ReelInVel<=0
    if time==0
        VelocityIC = GivenIC;
        Bool = 1;
    else
        Na = CurStepNumNodes;
        No = size(nodeVelocities,2);

        if PrevStepNumNodes==0
            Nc = CurStepNumNodes;
            Np = Nc;
        else
            Np = PrevStepNumNodes;
            Nc = CurStepNumNodes;
        end

        VelocityIC = [gndNodeVel(1)*ones(1,No-2);...
                      gndNodeVel(2)*ones(1,No-2);...
                      gndNodeVel(3)*ones(1,No-2)];
        if Nc == Np
            Bool = -1;
        else
            Bool = 1;
            VelocityIC(:,(No-Na+1):end) = nodeVelocities(:,(No-Na+2):end-1);
        end
    end         
else
    if time==0
        VelocityIC = GivenIC;
        Bool = 1;
    else
        Na = CurStepNumNodes;
        No = size(nodeVelocities,2);

        if PrevStepNumNodes==0
            Nc = CurStepNumNodes;
            Np = Nc;
        else
            Np = PrevStepNumNodes;
            Nc = CurStepNumNodes;
        end

        VelocityIC = [gndNodeVel(1)*ones(1,No-2);...
                      gndNodeVel(2)*ones(1,No-2);...
                      gndNodeVel(3)*ones(1,No-2)];
        if Nc == Np
            Bool = -1;
        else
            Bool = 1;
            linkVecs  = diff(nodeVelocities,1,2);
            linkVecsUnit = linkVecs./repmat(sqrt(sum((linkVecs.^2),1)),[3 1]);
            linkVecsUnit(isnan(linkVecsUnit))=0;
            VelocityIC(:,(No-Na+2):end) = nodeVelocities(:,(No-Na+3):end-1);
            VelocityIC(:,(No-Na+1)) = linkVecsUnit(:,(No-Na+1)).*ActiveLengths(:,No-Na+1);
        end
    end
end

== matlab function tetherM_cl/tetherM/MATLAB Function3 ==
  data: linkForceVecsPrev input; LA_Preserve output size=[1,thr.numNodes.Value-1]; nodePos input; nodeVel input; NumberNodesActive input; numNodes parameter; thrDiam parameter; youngsMod parameter; mass parameter; dampingRatio parameter
function LA_Preserve   = tetherNodeTensionForce(linkForceVecsPrev, nodePos, nodeVel, ...
    NumberNodesActive, numNodes, thrDiam, youngsMod, mass, dampingRatio)


No = numNodes;          %Total Nodes
Na = NumberNodesActive; %Nodes that arent reeled-in

%Finds Spring Constant
ZeroCheck = zeros(1,numNodes-1);
if Na>2
    ZeroCheck(1,(No-Na+1):end) = ones(1,Na-1);
end

%finds vectors between nodes
linkVecs  = diff(nodePos,1,2);
linkLength = sqrt(sum(linkVecs.^2));

%Finds unit vectors between nodes
linkUnitVecs = zeros(3,numNodes-1);
linkUnitVecs(1:3,(No-Na+1):end) = linkVecs(1:3,(No-Na+1):end)./repmat(sqrt(sum((linkVecs(1:3,(No-Na+1):end).^2),1)),[3 1]);

%prevent divide by zero if reeled in 
linkUnitVecs(isnan(linkUnitVecs))=0;

%Rate of change of all links
linkLengthDeriv = dot(nodeVel(:,2:end)-nodeVel(:,1:end-1),linkUnitVecs);

%Moves Reeled in bottom  node force to Ground Node
if ZeroCheck(1) == 0
    linkForceVecsPrev(:,1) = linkForceVecsPrev(:,No-Na+1);
    linkForceVecsPrev(:,No-Na+1) = 0;
end

W = youngsMod*(pi/4)*(thrDiam^2);
LA_Preserve = ((W.*(mass.*linkLengthDeriv.^2*dampingRatio.^2 + linkLength.*W + linkForceVecsPrev.*linkLength)).^(1/2) + linkLengthDeriv.*W.^(1/2).*dampingRatio.*mass.^(1/2)).^2./(linkForceVecsPrev + W).^2;

== matlab function tetherM_cl/tetherM/MATLAB Function4 ==
  data: OriginalLengths input; ActiveNodes output; ReeledOutLength input; TetherLength input; airNodePos input; midNodePos input; gndNodePos input; ReelInVel input; FirstLinkPrev input; ActiveLengths output size=[1,thr.numNodes.Value-1]; FirstLink output; minLinkLength parameter; minLinkDeviation parameter; Delta output; time input
function [ActiveNodes, ActiveLengths,FirstLink,Delta] = fcn(OriginalLengths, ReeledOutLength, TetherLength,airNodePos, midNodePos, gndNodePos,ReelInVel,FirstLinkPrev,minLinkLength, minLinkDeviation, time)

%Number of nodes
No = length(OriginalLengths)+1;

%Prealocated L and Activelengths
ActiveLengths = zeros(size(OriginalLengths));
L = zeros(size(ActiveLengths));

%Set Flags
flag = false;
flagOut1 = false;

%Set search parameter
a = No;
% if time==0
%     L = OriginalLengths;
%     FirstLink = L(1);
% else
    if ReeledOutLength == TetherLength  %Full Extension
        a = a+1;
        L(1:end) = OriginalLengths(1:end);
        FirstLink = OriginalLengths(1);
    elseif ReeledOutLength > TetherLength
        a = a+1;
        L(1:end) = OriginalLengths(1:end);
        FirstLink = OriginalLengths(1)+ReeledOutLength - TetherLength;
    else %Any amount of reel-in
        
        while flag == false %finds position of bottom link
            if ReeledOutLength == sum(OriginalLengths(a:end))
                flag = true;
            elseif ReeledOutLength < sum(OriginalLengths(a:end))+minLinkLength
                flag = true;
            else
                a=a-1;
            end
        end
        
        %Changing first link length
        FirstLink = OriginalLengths(a)-(sum(OriginalLengths((a):end))-ReeledOutLength);
        
        if FirstLink < minLinkLength %If below limit
            flagOut1  = true;
        end
        
        if a == No %If on last link
            L(end) = FirstLink;
        else
            if flagOut1==true %Min
                L((a):end)   = [FirstLink,OriginalLengths((a):end)];
            elseif flagOut1==false %Not min
                L((a):end) = [FirstLink,OriginalLengths((a+1):end)];
            end
        end
        
    end
% end

ActiveNodes = nnz(L)+1;
ActiveLengths = L;
Delta = a;

end
